simulink model "siWDqudong_FAN_MPC"  (R2024b)
settings: Solver=ode4  StartTime=0.0  StopTime=30  FixedStep=0.0005  RelTol=1e-3
undefined symbols (not defined in the file): MotorData, Q_beta_tune, Q_yaw_tune, R_alloc_tune, R_rate_tune, Road_Curvature_Map, Road_Mu_Map, Sim_Mu_Set, Sim_Vx_Set, Target_Speed_Map, W_util_tune
libraries: Solver_SF x1
(part 1 of 3)
Description:
  | V6 normalized model with fixed-speed PI torque demand. Created from V5; no implicit underspeed behavior in low-mu curves.
settings Model: SimulationMode=accelerator  Creator=zlm22  LastModifiedBy=zlm22
settings SolverCC: InsertRTBMode=Always
settings RTWCC: BuildConfiguration=Faster Runs

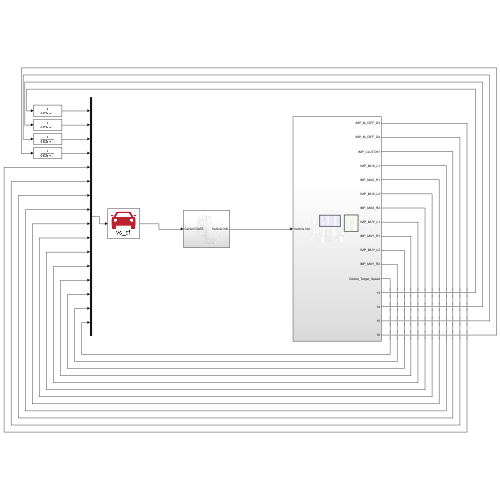
[thumbnail: Simulink's stored preview of the top-level diagram]
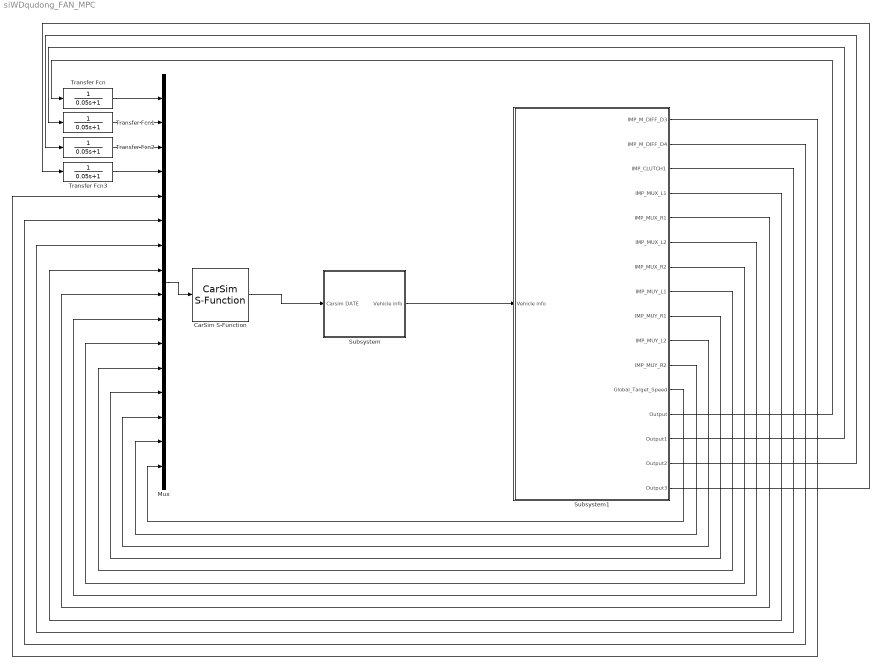
== system siWDqudong_FAN_MPC ==
  CarSim S-Function : Solver_SF/CarSim S-Function  Priority=1  SIMFILE=D:\Program Files (x86)\CarSim2024.1_DATA\simfile.sim  Run_RTs=off  vs_state_ind=Run  StopMode_ind=Vehicle Model
  Mux : Mux  Inputs=16
  Subsystem : Subsystem
  Subsystem1 : Subsystem
  Transfer Fcn{,1..3} (4 alike) : TransferFcn  Denominator=[0.05 1]
  wires:
  Transfer Fcn/1 -> Mux/1
  Transfer Fcn1/1 -> Mux/2
  Transfer Fcn2/1 -> Mux/3
  Transfer Fcn3/1 -> Mux/4
  Subsystem/1(Vehicle info) -> Subsystem1/1(Vehicle info)
  Subsystem1/1(IMP_M_DIFF_D3) -> Mux/5
  Subsystem1/2(IMP_M_DIFF_D4) -> Mux/6
  Subsystem1/3(IMP_CLUTCH1) -> Mux/7
  Subsystem1/4(IMP_MUX_L1) -> Mux/8
  Subsystem1/5(IMP_MUX_R1) -> Mux/9
  Subsystem1/6(IMP_MUX_L2) -> Mux/10
  Subsystem1/7(IMP_MUX_R2) -> Mux/11
  Subsystem1/8(IMP_MUY_L1) -> Mux/12
  Subsystem1/9(IMP_MUY_R1) -> Mux/13
  Subsystem1/10(IMP_MUY_L2) -> Mux/14
  Subsystem1/11(IMP_MUY_R2) -> Mux/15
  Subsystem1/12(Global_Target_Speed) -> Mux/16
  Subsystem1/13(Output) -> Transfer Fcn/1
  Subsystem1/14(Output1) -> Transfer Fcn1/1
  Subsystem1/15(Output2) -> Transfer Fcn2/1
  Subsystem1/16(Output3) -> Transfer Fcn3/1
  Mux/1 -> CarSim S-Function/1
  CarSim S-Function/1 -> Subsystem/1(Carsim DATE)

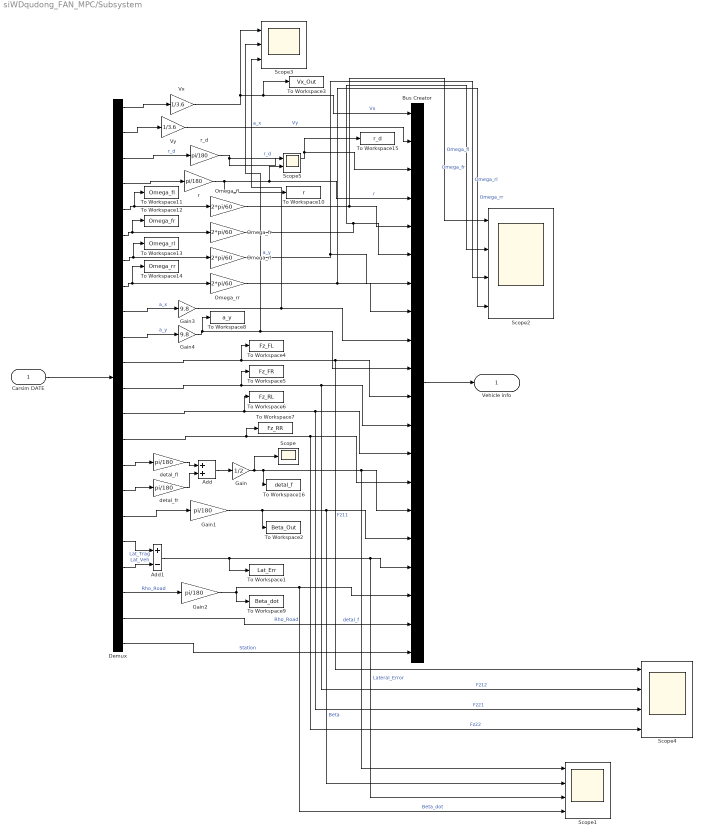
== system siWDqudong_FAN_MPC/Subsystem ==
  Carsim DATE : Inport
  Add : Sum
  Add1 : Sum  Inputs=+-
  Bus Creator : BusCreator  Inputs=20
  Demux : Demux  Outputs=22
  Gain : Gain  Gain=1/2
  Gain1 : Gain  Gain=pi/180
  Gain2 : Gain  Gain=pi/180
  Gain3 : Gain  Gain=9.8
  Gain4 : Gain  Gain=9.8
  Omega_fl : Gain  Gain=2*pi/60
  Omega_fr : Gain  Gain=2*pi/60
  Omega_rl : Gain  Gain=2*pi/60
  Omega_rr : Gain  Gain=2*pi/60
  Scope : Scope
  Scope1 : Scope  NumInputPorts=4
  Scope2 : Scope  NumInputPorts=4
  Scope3 : Scope  NumInputPorts=3
  Scope4 : Scope  NumInputPorts=4
  Scope5 : Scope  NumInputPorts=2
  To Workspace1 : ToWorkspace  VariableName=Lat_Err  SampleTime=-1
  To Workspace10 : ToWorkspace  VariableName=r  SampleTime=-1
  To Workspace11 : ToWorkspace  VariableName=Omega_fl  SampleTime=-1
  To Workspace12 : ToWorkspace  VariableName=Omega_fr  SampleTime=-1
  To Workspace13 : ToWorkspace  VariableName=Omega_rl  SampleTime=-1
  To Workspace14 : ToWorkspace  VariableName=Omega_rr  SampleTime=-1
  To Workspace15 : ToWorkspace  VariableName=r_d  SampleTime=-1
  To Workspace16 : ToWorkspace  VariableName=detal_f  SampleTime=-1
  To Workspace2 : ToWorkspace  VariableName=Beta_Out  SampleTime=-1
  To Workspace3 : ToWorkspace  VariableName=Vx_Out  SampleTime=-1
  To Workspace4 : ToWorkspace  VariableName=Fz_FL  SaveFormat=Timeseries  SampleTime=-1
  To Workspace5 : ToWorkspace  VariableName=Fz_FR  SaveFormat=Timeseries  SampleTime=-1
  To Workspace6 : ToWorkspace  VariableName=Fz_RL  SaveFormat=Timeseries  SampleTime=-1
  To Workspace7 : ToWorkspace  VariableName=Fz_RR  SaveFormat=Timeseries  SampleTime=-1
  To Workspace8 : ToWorkspace  VariableName=a_y  SampleTime=-1
  To Workspace9 : ToWorkspace  VariableName=Beta_dot  SampleTime=-1
  Vx : Gain  Gain=1/3.6
  Vy : Gain  Gain=1/3.6
  detal_fl : Gain  Gain=pi/180
  detal_fr : Gain  Gain=pi/180
  r : Gain  Gain=pi/180
  r_d : Gain  Gain=pi/180
  Vehicle info : Outport
  wires:
  Demux/3 -> r_d/1  "r_d"
  Demux/11 -> To Workspace4/1, Scope4/1, Bus Creator/11  "Fz11"
  Demux/8 -> To Workspace14/1, Omega_rr/1
  Vy/1 -> Bus Creator/2  "Vy"
  Demux/7 -> To Workspace13/1, Omega_rl/1
  Demux/14 -> To Workspace7/1, Scope4/4, Bus Creator/14  "Fz22"
  Demux/4 -> r/1
  Demux/5 -> To Workspace11/1, Omega_fl/1
  Demux/13 -> To Workspace6/1, Scope4/3, Bus Creator/13  "Fz21"
  Omega_rl/1 -> Scope2/3, Bus Creator/7  "Omega_rl"
  Demux/12 -> To Workspace5/1, Scope4/2, Bus Creator/12  "Fz12"
  Demux/16 -> detal_fr/1
  Omega_fr/1 -> Scope2/2, Bus Creator/6  "Omega_fr"
  Demux/6 -> To Workspace12/1, Omega_fr/1
  Demux/15 -> detal_fl/1
  Vx/1 -> Scope3/1, To Workspace3/1, Bus Creator/1  "Vx"
  r/1 -> Scope5/2, Bus Creator/4, To Workspace10/1  "r"
  Bus Creator/1 -> Vehicle info/1
  Omega_fl/1 -> Scope2/1, Bus Creator/5  "Omega_fl"
  Omega_rr/1 -> Scope2/4, Bus Creator/8  "Omega_rr"
  Demux/10 -> Gain4/1  "a_y"
  Demux/9 -> Gain3/1  "a_x"
  detal_fr/1 -> Add/2
  detal_fl/1 -> Add/1
  Add/1 -> Gain/1
  Gain/1 -> Scope/1, To Workspace16/1, Scope1/1, Bus Creator/15  "detal_f"
  Demux/1 -> Vx/1
  Demux/2 -> Vy/1
  Demux/17 -> Gain1/1
  Gain1/1 -> To Workspace2/1, Bus Creator/16, Scope1/2  "Beta"
  Gain2/1 -> Scope1/4, Bus Creator/18, To Workspace9/1  "Beta_dot"
  r_d/1 -> To Workspace15/1, Bus Creator/3, Scope5/1  "r_d"
  Carsim DATE/1 -> Demux/1
  Gain4/1 -> To Workspace8/1, Scope3/2, Bus Creator/10  "a_y"
  Gain3/1 -> Scope3/3, Bus Creator/9  "a_x"
  Demux/22 -> Bus Creator/20  "Station"
  Demux/21 -> Bus Creator/19  "Rho_Road"
  Demux/20 -> Gain2/1  "Rho_Road"
  Demux/18 -> Add1/1  "Lat_Trag"
  Demux/19 -> Add1/2  "Lat_Veh"
  Add1/1 -> To Workspace1/1, Scope1/3, Bus Creator/17  "Lateral_Error"

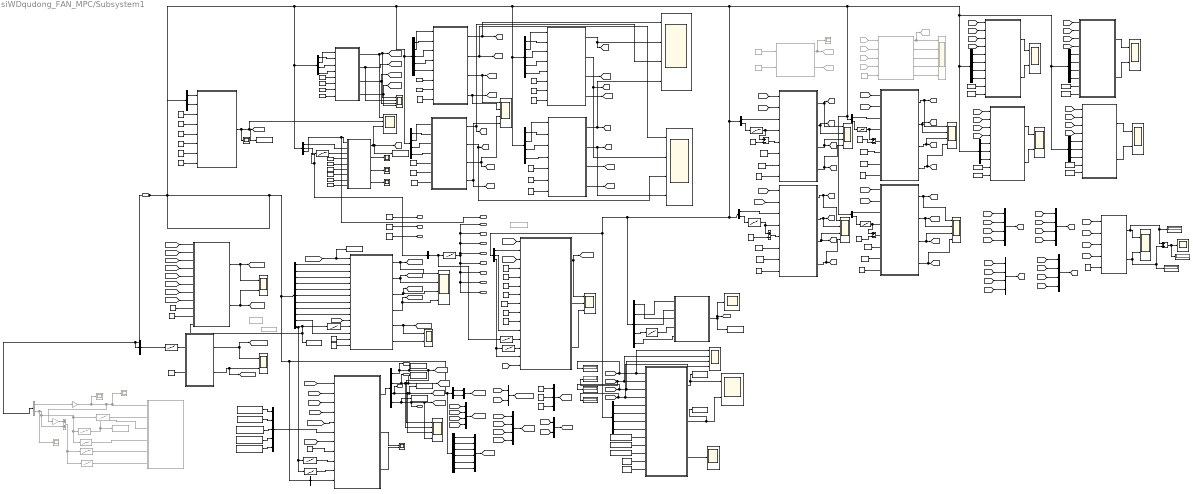
== system siWDqudong_FAN_MPC/Subsystem1 ==
  note: E_total_kWh
  note: Subsystem3
  note: 轮胎力
  Vehicle info : Inport
  Add1 : Sum
  Add{2..4,6} (4 alike) : Sum  Inputs=+-
  Add5 : Sum  Commented=on
  Bus Creator : BusCreator  Inputs=6
  Bus Creator1 : BusCreator  Inputs=2
  Bus Selector : BusSelector  OutputSignals=Omega_fl,Omega_fr,Omega_rl,Omega_rr,Fz11,Fz12,Fz21,Fz22,a_y,Lateral_Error,Station
  Bus Selector1 : BusSelector  OutputSignals=Vx,detal_f,Fz11,Fz12,Fz21,Fz22
  Bus Selector10 : BusSelector  OutputSignals=Fz11,Station
  Bus Selector11 : BusSelector  OutputSignals=Fz21,Station
  Bus Selector12 : BusSelector  OutputSignals=Fz12,Station
  Bus Selector13 : BusSelector  OutputSignals=Fz22,Station
  Bus Selector15 : BusSelector  Commented=on  OutputSignals=Vx,Station
  Bus Selector16 : BusSelector  OutputSignals=detal_f
  Bus Selector17 : BusSelector  OutputSignals=Vx,Vy,r_d,detal_f
  Bus Selector19 : BusSelector  OutputSignals=Vx,Vy,r_d,detal_f
  Bus Selector2 : BusSelector  OutputSignals=Beta,r_d
  Bus Selector20 : BusSelector  OutputSignals=Vx,Vy,r_d
  Bus Selector21 : BusSelector  OutputSignals=Vx,Vy,r_d
  Bus Selector22 : BusSelector  OutputSignals=Station
  Bus Selector23 : BusSelector  OutputSignals=detal_f,Station,Vx
  Bus Selector24 : BusSelector  OutputSignals=Station
  Bus Selector25 : BusSelector  OutputSignals=Omega_fl,Omega_fr,Omega_rl,Omega_rr
  Bus Selector26 : BusSelector  OutputSignals=Vx,detal_f,Beta
  Bus Selector27 : BusSelector  OutputSignals=Vx,Beta,Beta_dot,Station,detal_f
  Bus Selector3 : BusSelector  OutputSignals=Vx,detal_f
  Bus Selector5 : BusSelector  OutputSignals=Vy,Vx,r_d,Omega_fl,detal_f
  Bus Selector6 : BusSelector  OutputSignals=Vy,Vx,r_d,detal_f
  Bus Selector7 : BusSelector  OutputSignals=Vy,Vx,r_d,Omega_fr,detal_f
  Bus Selector8 : BusSelector  OutputSignals=Vy,Vx,r_d,Omega_rl
  Bus Selector9 : BusSelector  OutputSignals=Vy,Vx,r_d,Omega_rr
  Constant{1,7,18,21,30,48,90} (7 alike) : Constant  Value=1.152
  Constant{2,8,10,13,49,93,95} (7 alike) : Constant  Value=1.528
  Constant{9,11,14,16..17,19,78,92,94,96} (10 alike) : Constant  Value=1.565
  Constant{12,15,20,22,54} (5 alike) : Constant  Value=0.347
  Constant{23..25,60,82} (5 alike) : Constant  Value=0
  Constant{26,73,81,84,91} (5 alike) : Constant  Value=0.05
  Constant27 : Constant  Commented=on  Value=3
  Constant28 : Constant  Commented=on  Value=0.001
  Constant{29,32,35,38} (4 alike) : Constant  Value=0.6
  Constant{3,31,37,50,79} (5 alike) : Constant  Value=63833
  Constant33 : Constant  Value=44230
  Constant{4,34,40,51,88} (5 alike) : Constant  Value=48729
  Constant36 : Constant  Value=57917
  Constant39 : Constant  Value=44230
  Constant41 : Constant  Commented=on  Value=0.347
  Constant{6,42,59,86,97} (5 alike) : Constant  Value=0.01
  Constant43 : Constant  Value=800
  Constant44 : Constant  Commented=on  Value=Sim_Mu_Set
  Constant45 : Constant  Value=MotorData.Speed_Axis
  Constant47 : Constant  Value=1810
  Constant5 : Constant  Value=1810
  Constant52 : Constant  Value=9.81
  Constant53 : Constant  Value=MotorData.Torque_Axis
  Constant55 : Constant  Value=1810
  Constant56 : Constant  Value=9.81
  Constant57 : Constant  Value=45
  Constant58 : Constant  Value=5.0
  Constant63 : Constant  Value=Q_beta_tune
  Constant64 : Constant  Value=Q_yaw_tune
  Constant66 : Constant  Commented=on  Value=Sim_Vx_Set
  Constant68 : Constant  Commented=on  Value=Sim_Vx_Set
  Constant69 : Constant  Value=R_alloc_tune
  Constant71 : Constant  Value=R_rate_tune
  Constant72 : Constant  Value=W_util_tune
  Constant77 : Constant  Value=MotorData.Eff_Map
  Constant80 : Constant  Value=0.005
  Constant89 : Constant  Value=57917
  Demux : Demux
  Display{,1..6} (7 alike) : Display
  From68 : From  Commented=on  GotoTag=Fx_fl
  From69 : From  Commented=on  GotoTag=Fx_fr
  From70 : From  Commented=on  GotoTag=Fx_rl
  From71 : From  Commented=on  GotoTag=Fx_rr
  Gain : Gain  Commented=on  Gain=3.6
  Gain2 : Gain  Commented=on  Gain=1.2
  Goto29 : Goto  Commented=on  GotoTag=mu_y
  Goto5 : Goto  Commented=on  GotoTag=mu_x
  MATLAB Function : MATLAB Function  TreatAsAtomicUnit=on  SystemSampleTime=0.01
  MATLAB Function1 : MATLAB Function  TreatAsAtomicUnit=on
  MATLAB Function10 : MATLAB Function  TreatAsAtomicUnit=on
  MATLAB Function14 : MATLAB Function  Commented=on  TreatAsAtomicUnit=on
  MATLAB Function15 : MATLAB Function  TreatAsAtomicUnit=on  SystemSampleTime=0.01
  MATLAB Function16 : MATLAB Function  TreatAsAtomicUnit=on
  MATLAB Function17 : MATLAB Function  TreatAsAtomicUnit=on
  MATLAB Function18 : MATLAB Function  TreatAsAtomicUnit=on
  MATLAB Function19 : MATLAB Function  TreatAsAtomicUnit=on  SystemSampleTime=0.01
  MATLAB Function2 : MATLAB Function  TreatAsAtomicUnit=on  SystemSampleTime=0.01
  MATLAB Function20 : MATLAB Function  Commented=on  TreatAsAtomicUnit=on
  MATLAB Function21 : MATLAB Function  TreatAsAtomicUnit=on  SystemSampleTime=0.01
  MATLAB Function22 : MATLAB Function  TreatAsAtomicUnit=on
  MATLAB Function23 : MATLAB Function  TreatAsAtomicUnit=on  SystemSampleTime=0.01
  MATLAB Function24 : MATLAB Function  TreatAsAtomicUnit=on
  MATLAB Function25 : MATLAB Function  TreatAsAtomicUnit=on
  MATLAB Function3 : MATLAB Function  TreatAsAtomicUnit=on  SystemSampleTime=0.01
  MATLAB Function4 : MATLAB Function  TreatAsAtomicUnit=on
  MATLAB Function5 : MATLAB Function  TreatAsAtomicUnit=on
  MATLAB Function6 : MATLAB Function  TreatAsAtomicUnit=on
  MATLAB Function7 : MATLAB Function  TreatAsAtomicUnit=on
  MATLAB Function8 : MATLAB Function  TreatAsAtomicUnit=on
  MATLAB Function9 : MATLAB Function  TreatAsAtomicUnit=on
  MU : Lookup_n-D  Commented=on  NumberOfTableDimensions=1  BreakpointsForDimension1=Road_Mu_Map(:, 1)  Table=Road_Mu_Map(:, 2)  InternalRulePriority=Speed  RndMeth=Simplest
  Mu12 : Lookup_n-D  Commented=on  NumberOfTableDimensions=1  BreakpointsForDimension1=Road_Mu_Map(:, 1)  Table=Road_Mu_Map(:, 2)  InternalRulePriority=Speed  RndMeth=Simplest
  Mu{2..9,13..14} (10 alike) : Lookup_n-D  NumberOfTableDimensions=1  BreakpointsForDimension1=Road_Mu_Map(:, 1)  Table=Road_Mu_Map(:, 2)  InternalRulePriority=Speed  RndMeth=Simplest
  Mux : Mux  Inputs=2
  Mux{1,5..9} (6 alike) : Mux
  Mux10 : Mux  Inputs=5
  Mux2 : Mux  Inputs=2
  Mux4 : Mux  Inputs=3
  Radius1 : Lookup_n-D  Commented=on  NumberOfTableDimensions=1  BreakpointsForDimension1=Road_Curvature_Map(:, 1)  Table=Road_Curvature_Map(:, 2)  InternalRulePriority=Speed  RndMeth=Simplest
  Radius2 : Lookup_n-D  Commented=on  NumberOfTableDimensions=1  BreakpointsForDimension1=Road_Curvature_Map(:, 1)  Table=Road_Curvature_Map(:, 2)  InternalRulePriority=Speed  RndMeth=Simplest
  Radius3 : Lookup_n-D  NumberOfTableDimensions=1  BreakpointsForDimension1=Road_Curvature_Map(:, 1)  Table=Road_Curvature_Map(:, 2)  InternalRulePriority=Speed  RndMeth=Simplest
  Radius4 : Lookup_n-D  NumberOfTableDimensions=1  BreakpointsForDimension1=Road_Curvature_Map(:, 1)  Table=Road_Curvature_Map(:, 2)  InternalRulePriority=Speed  RndMeth=Simplest
  SI : Scope
  Scope{,1..2,5,10..14,45} (10 alike) : Scope  NumInputPorts=2
  Scope{3..4,6,9,15..18,20,28,30,48} (12 alike) : Scope  NumInputPorts=4
  Scope{8,21..22,47} (4 alike) : Scope  Commented=on
  Scope{23,32..34,44,49} (6 alike) : Scope
  Scope24 : Scope  Commented=on  NumInputPorts=5
  Scope7 : Scope  NumInputPorts=3
  T_max : Constant  Value=800
  T_min : Constant  Value=-200
  To Workspace : ToWorkspace  VariableName=SI_Out  SaveFormat=Timeseries  SampleTime=-1
  To Workspace10 : ToWorkspace  VariableName=R_ref  SampleTime=-1
  To Workspace12 : ToWorkspace  VariableName=beta_ref  SampleTime=-1
  To Workspace13 : ToWorkspace  VariableName=Sim_Station  SampleTime=-1
  To Workspace14 : ToWorkspace  Commented=on  VariableName=Mu  SampleTime=-1
  To Workspace3 : ToWorkspace  VariableName=Total_Power_Out  SampleTime=-1
  To Workspace4 : ToWorkspace  VariableName=Motor_Torque_FL  SampleTime=-1
  To Workspace5 : ToWorkspace  VariableName=Motor_Torque_FR  SampleTime=-1
  To Workspace6 : ToWorkspace  VariableName=Motor_Torque_RL  SampleTime=-1
  To Workspace7 : ToWorkspace  VariableName=Motor_Torque_RR  SampleTime=-1
  To Workspace8 : ToWorkspace  VariableName=E_total_kWh  SampleTime=-1
  To Workspace9 : ToWorkspace  VariableName=P_total_kW  SampleTime=-1
  Vx1 : Lookup_n-D  NumberOfTableDimensions=1  BreakpointsForDimension1=Target_Speed_Map(:, 1)  Table=Target_Speed_Map(:, 2)  InternalRulePriority=Speed  RndMeth=Simplest
  Vx2 : Lookup_n-D  Commented=on  NumberOfTableDimensions=1  BreakpointsForDimension1=Target_Speed_Map(:, 1)  Table=Target_Speed_Map(:, 2)  InternalRulePriority=Speed  RndMeth=Simplest
  delta_T_max : Constant  Value=2000
  unitire轮胎力 : MATLAB Function  TreatAsAtomicUnit=on
  侧偏角计算 : MATLAB Function  TreatAsAtomicUnit=on
  总需求扭矩 : Goto  Commented=on  GotoTag=Td
  横纵向附着系数 : MATLAB Function  Commented=on  TreatAsAtomicUnit=on
  IMP_M_DIFF_D3 : Outport
  IMP_M_DIFF_D4 : Outport  Port=2
  IMP_CLUTCH1 : Outport  Port=3
  IMP_MUX_L1 : Outport  Port=4
  IMP_MUX_R1 : Outport  Port=5
  IMP_MUX_L2 : Outport  Port=6
  IMP_MUX_R2 : Outport  Port=7
  IMP_MUY_L1 : Outport  Port=8
  IMP_MUY_R1 : Outport  Port=9
  IMP_MUY_L2 : Outport  Port=10
  IMP_MUY_R2 : Outport  Port=11
  Global_Target_Speed : Outport  Port=12
  Output : Outport  Port=13
  Output1 : Outport  Port=14
  Output2 : Outport  Port=15
  Output3 : Outport  Port=16
  wires:
  MATLAB Function5/1(Sx_fr) -> [Sx_fr], Scope9/2
  Bus Selector7/1 -> MATLAB Function5/2(Vy)  "<Vy>"
  Constant13/1 -> MATLAB Function7/5(lr)
  Constant21/1 -> MATLAB Function5/6(lf)
  MATLAB Function8/3(Fbar_x_rl) -> Scope17/3, [Fsx_rl]
  MATLAB Function6/1(Sx_rl) -> [Sx_rl], Scope9/3
  Constant14/1 -> MATLAB Function7/6(twr)
  MATLAB Function7/1(Sx_rr) -> [Sx_rr], Scope9/4
  Constant1/1 -> MATLAB Function4/3(lf)
  Bus Selector11/1 -> MATLAB Function8/3(Fz_rl)  "<Fz21>"
  MATLAB Function9/2(Fy_fr) -> Scope15/2, [Fy_fr]
  Bus Selector6/4 -> 侧偏角计算/4(delta_f_rad)  "<detal_f>"
  MATLAB Function5/2(Sy_fr) -> [Sy_fr], Scope28/2
  Constant47/1 -> MATLAB Function17/4(m)
  Bus Selector5/5 -> unitire轮胎力/5(delta_f)  "<detal_f>"
  [Sx_fr] -> MATLAB Function9/1(Sx_fr)
  Constant52/1 -> MATLAB Function17/9(g)
  MATLAB Function17/1(r_d) -> [r_d], To Workspace10/1, Scope30/3  "r_ref"
  Constant15/1 -> MATLAB Function7/7(Re)
  MATLAB Function9/1(Fx_fr) -> Scope15/1, [Fx_fr]
  MATLAB Function10/1(Fx_rr) -> Scope18/1, [Fx_rr]
  MATLAB Function1/1(Fx_fl) -> [Fx_fl], Scope48/1
  MATLAB Function7/2(Sy_rr) -> Scope28/4, [Sy_rr]
  Constant2/1 -> MATLAB Function4/4(lr)
  MATLAB Function20/1(Td) -> Scope24/1, 总需求扭矩/1
  Constant38/1 -> MATLAB Function10/8(E)
  [Sy_fr] -> MATLAB Function9/2(Sy_fr)
  Constant9/1 -> 侧偏角计算/7(twf)
  Bus Selector10/1 -> MATLAB Function1/3(Fz_fl)  "<Fz11>"
  Bus Selector7/4 -> MATLAB Function5/4(omega_fr)  "<Omega_fr>"
  Constant4/1 -> MATLAB Function4/6(Kyr)
  Constant5/1 -> MATLAB Function4/7(m)
  Constant8/1 -> 侧偏角计算/6(lr)
  Constant27/1 -> 横纵向附着系数/1(road_condition)
  Bus Selector3/2 -> MATLAB Function4/2(delta_f)  "<detal_f>"
  Bus Selector3/1 -> MATLAB Function4/1(Vx)  "<Vx>"
  Constant6/1 -> MATLAB Function4/8(dt)
  Constant17/1 -> MATLAB Function5/7(twf)
  MATLAB Function4/1(beta_ref) -> Scope44/1, To Workspace12/1, [beta_ref], Scope30/2  "beta_ref"
  MATLAB Function1/3(Fbar_x_fl) -> Scope48/3, [Fsx_fl]
  Constant48/1 -> MATLAB Function17/5(lf)
  Constant3/1 -> MATLAB Function4/5(Kyf)
  MATLAB Function1/4(Fbar_y_fl) -> Scope48/4, [Fsy_fl]
  Constant29/1 -> MATLAB Function1/8(E)
  From68/1 -> MATLAB Function20/1(Fx_fl)
  Bus Selector8/4 -> MATLAB Function6/4(omega_rl)  "<Omega_rl>"
  MATLAB Function6/2(Sy_rl) -> Scope28/3, [Sy_rl]
  From71/1 -> MATLAB Function20/4(Fx_rr)
  Constant50/1 -> MATLAB Function17/7(Kf0)
  Bus Selector5/4 -> unitire轮胎力/4(omega_fl)  "<Omega_fl>"
  Bus Selector6/1 -> 侧偏角计算/2(Vy)  "<Vy>"
  Constant49/1 -> MATLAB Function17/6(lr)
  MATLAB Function8/4(Fbar_y_rl) -> Scope17/4, [Fsy_rl]
  MATLAB Function9/4(Fbar_y_fr) -> Scope15/4, [Fsy_fr]
  Constant51/1 -> MATLAB Function17/8(Kr0)
  MATLAB Function17/4(r_limit) -> Scope34/1
  MATLAB Function17/2(K_s) -> Scope32/1
  MATLAB Function17/3(r_ideal) -> Scope33/1
  Constant22/1 -> MATLAB Function5/8(Re)
  横纵向附着系数/1(mu_x) -> Scope47/1, Goto5/1
  Bus Selector12/1 -> MATLAB Function9/3(Fz_fr)  "<Fz12>"
  [Sx_fl] -> MATLAB Function1/1(Sx_fl)
  Bus Selector9/4 -> MATLAB Function7/4(omega_rr)  "<Omega_rr>"
  unitire轮胎力/1(Sx_fl) -> Scope9/1, [Sx_fl]
  From69/1 -> MATLAB Function20/2(Fx_fr)
  From70/1 -> MATLAB Function20/3(Fx_rl)
  Constant10/1 -> MATLAB Function6/5(lr)
  [Sy_rr] -> MATLAB Function10/2(Sy_rr)
  Constant41/1 -> MATLAB Function20/5(r_e)
  Constant35/1 -> MATLAB Function9/8(E)
  [Sy_rl] -> MATLAB Function8/2(Sy_rl)
  Constant7/1 -> 侧偏角计算/5(lf)
  MATLAB Function9/3(Fbar_x_fr) -> Scope15/3, [Fsx_fr]
  Bus Selector13/1 -> MATLAB Function10/3(Fz_rr)  "<Fz22>"
  MATLAB Function1/2(Fy_fl) -> [Fy_fl], Scope48/2
  MATLAB Function10/4(Fbar_y_rr) -> Scope18/4, [Fsy_rr]
  MATLAB Function10/2(Fy_rr) -> Scope18/2, [Fy_rr]
  MATLAB Function10/3(Fbar_x_rr) -> Scope18/3, [Fsx_rr]
  Mu5/1 -> Add6/1, MATLAB Function1/4(mu_x)
  [Sx_rr] -> MATLAB Function10/1(Sx_rr)
  Constant32/1 -> MATLAB Function8/8(E)
  MATLAB Function8/1(Fx_rl) -> Scope17/1, [Fx_rl]
  MATLAB Function8/2(Fy_rl) -> Scope17/2, [Fy_rl]
  [Sy_fl] -> MATLAB Function1/2(Sy_fl)
  Constant19/1 -> unitire轮胎力/7(twf)
  [Sx_rl] -> MATLAB Function8/1(Sx_rl)
  横纵向附着系数/2(mu_y) -> Goto29/1
  Constant28/1 -> 横纵向附着系数/2(slip_ratio)
  Bus Selector9/1 -> MATLAB Function7/2(Vy)  "<Vy>"
  Constant18/1 -> unitire轮胎力/6(lf)
  unitire轮胎力/2(Sy_fl) -> Scope28/1, [Sy_fl]
  Constant16/1 -> 侧偏角计算/8(twr)
  Constant11/1 -> MATLAB Function6/6(twr)
  Bus Selector8/1 -> MATLAB Function6/2(Vy)  "<Vy>"
  Constant20/1 -> unitire轮胎力/8(Re)
  Bus Selector5/1 -> unitire轮胎力/2(Vy)  "<Vy>"
  Vehicle info/1 -> Bus Selector/1, Bus Selector2/1, Bus Selector1/1, Bus Selector16/1, Bus Selector23/1, Bus Selector6/1, Bus Selector9/1, Bus Selector7/1, Bus Selector10/1, Bus Selector27/1, Bus Selector25/1, Bus Selector26/1, Bus Selector11/1, Bus Selector21/1, Bus Selector19/1, Bus Selector20/1, Bus Selector17/1, Bus Selector13/1, Bus Selector12/1, Bus Selector8/1, Bus Selector5/1, Bus Selector3/1, Bus Selector15/1, Bus Selector24/1
  MATLAB Function20/5(T_rr) -> Scope24/5
  MATLAB Function20/4(T_rl) -> Scope24/4
  MATLAB Function20/3(T_fr) -> Scope24/3
  MATLAB Function20/2(T_fl) -> Scope24/2
  [T_ZY_RR] -> Display3/1, MATLAB Function2/4(T_rr), Scope6/4
  [T_ZY_RL] -> Display2/1, Scope6/3, MATLAB Function2/3(T_rl)
  [T_ZY_FL] -> Display/1, MATLAB Function2/1(T_fl), Scope6/1
  [T_ZY_FR] -> Display1/1, MATLAB Function2/2(T_fr), Scope6/2
  Bus Selector25/1 -> MATLAB Function2/5(w_fl)  "<Omega_fl>"
  Bus Selector25/2 -> MATLAB Function2/6(w_fr)  "<Omega_fr>"
  Bus Selector25/3 -> MATLAB Function2/7(w_rl)  "<Omega_rl>"
  MATLAB Function2/3(P_avg_kW) -> Scope49/1
  Constant55/1 -> MATLAB Function15/4(m)
  Constant56/1 -> MATLAB Function15/5(g)
  MATLAB Function15/1(T_total) -> [T_total], Scope7/1
  MATLAB Function18/1(Vx_safe_cmd) -> Scope45/1, [Vx_safe_cmd]
  MATLAB Function18/2(Ax_cmd_final) -> Scope45/2, [Ax_cmd_final]
  [Vx_safe_cmd] -> MATLAB Function15/1(Vx_cmd)
  [Ax_cmd_final] -> MATLAB Function15/3(Ax_cmd)
  MATLAB Function2/2(E_total_kWh) -> To Workspace8/1, Scope2/2
  MATLAB Function2/1(P_total_kW) -> To Workspace9/1, Scope2/1
  Constant73/1 -> MATLAB Function18/2(dt)
  Bus Selector27/3 -> MATLAB Function19/2(Beta_dot)  "<Beta_dot>"
  MATLAB Function19/1(SI_Out) -> To Workspace/1, SI/1, [SI]  "SI_Out"
  [Fy_fl] -> MATLAB Function23/1(Fy_fl)
  [Fy_fr] -> MATLAB Function23/2(Fy_fr)
  [Fy_rl] -> MATLAB Function23/3(Fy_rl)
  [Fy_rr] -> MATLAB Function23/4(Fy_rr)
  [alpha_fl] -> MATLAB Function23/5(Alpha_fl)
  [alpha_fr] -> MATLAB Function23/6(Alpha_fr)
  [alpha_rl] -> MATLAB Function23/7(Alpha_rl)
  [alpha_rr] -> MATLAB Function23/8(Alpha_rr)
  Constant88/1 -> MATLAB Function23/10(Cr0)
  Constant79/1 -> MATLAB Function23/9(Cf0)
  MATLAB Function23/1(Cf_eq) -> Scope5/1, [Cf_eq]
  MATLAB Function23/2(Cr_eq) -> Scope5/2, [Cr_eq]
  Constant23/1 -> IMP_M_DIFF_D3/1
  Constant24/1 -> IMP_M_DIFF_D4/1
  Constant25/1 -> IMP_CLUTCH1/1
  Mu3/1 -> IMP_MUX_R2/1, IMP_MUX_L2/1, IMP_MUX_R1/1, IMP_MUX_L1/1, IMP_MUY_L1/1, IMP_MUY_R1/1, IMP_MUY_L2/1, IMP_MUY_R2/1
  Constant81/1 -> Add2/2
  Constant84/1 -> Add3/2
  Add4/1 -> MATLAB Function8/5(mu_y)
  Mu7/1 -> MATLAB Function8/4(mu_x), Add4/1
  Constant91/1 -> Add4/2
  [T_total] -> To Workspace3/1, MATLAB Function3/1(T_total_req)
  Bus Selector/8 -> MATLAB Function3/9(Fz_rr)  "<Fz22>"
  Bus Selector/7 -> MATLAB Function3/8(Fz_rl)  "<Fz21>"
  Bus Selector/6 -> MATLAB Function3/7(Fz_fr)  "<Fz12>"
  Bus Selector/5 -> MATLAB Function3/6(Fz_fl)  "<Fz11>"
  Bus Selector/4 -> MATLAB Function3/5(w_rr)  "<Omega_rr>"
  Bus Selector/3 -> MATLAB Function3/4(w_rl)  "<Omega_rl>"
  Bus Selector/2 -> MATLAB Function3/3(w_fr)  "<Omega_fr>"
  Bus Selector/1 -> MATLAB Function3/2(w_fl)  "<Omega_fl>"
  Constant43/1 -> MATLAB Function3/14(T_motor_max)
  MATLAB Function3/5(Mode_Out) -> Scope/1, [Mode_Signal]
  MATLAB Function3/1(T_ref_fl) -> [T_ref_fl], Scope4/1
  MATLAB Function3/2(T_ref_fr) -> [T_ref_fr], Scope4/2
  MATLAB Function3/3(T_ref_rl) -> [T_ref_rl], Scope4/3
  MATLAB Function3/4(T_ref_rr) -> [T_ref_rr], Scope4/4
  Constant42/1 -> MATLAB Function3/15(dt)
  [beta_ref] -> Mux/1
  [r_d] -> Mux/2
  [T_ref_fl] -> Mux1/1
  [T_ref_fr] -> Mux1/2
  [T_ref_rl] -> Mux1/3
  [T_ref_rr] -> Mux1/4
  Mux1/1 -> [T_ref_upper]
  [Cf_eq] -> Mux2/1
  [Cr_eq] -> Mux2/2
  Mux2/1 -> [Stiffness_Input]
  Bus Selector1/3 -> Bus Creator/3  "<Fz11>"
  Bus Selector1/4 -> Bus Creator/4  "<Fz12>"
  Bus Selector1/5 -> Bus Creator/5  "<Fz21>"
  Bus Selector1/6 -> Bus Creator/6  "<Fz22>"
  Bus Creator/1 -> [Vehicle_State]
  Bus Selector2/1 -> Bus Creator1/1  "<Beta>"
  Bus Selector2/2 -> Bus Creator1/2  "<r_d>"
  Bus Creator1/1 -> [x_curr]
  T_min/1 -> Mux4/1
  T_max/1 -> Mux4/2
  delta_T_max/1 -> Mux4/3
  Mux4/1 -> [Constraints]
  [x_curr] -> MATLAB Function/1(x_curr)
  [x_ref] -> MATLAB Function/2(x_ref)
  [T_ref_upper] -> MATLAB Function/3(T_ref_upper_in)
  [Vehicle_State] -> MATLAB Function/4(Vehicle_State)
  [Stiffness_Input] -> MATLAB Function/5(Stiffness_Input)
  [Constraints] -> MATLAB Function/7(Constraints)
  MATLAB Function/2(Solver_Status) -> Scope1/1
  MATLAB Function/3(Debug_Info) -> Scope1/2
  MATLAB Function/1(T_final_opt) -> Demux/1
  Demux/1 -> Output/1, To Workspace4/1, [T_ZY_FL], Scope3/1  "F11"
  Demux/2 -> Output1/1, To Workspace5/1, [T_ZY_FR], Scope3/2  "F12"
  Demux/3 -> Output2/1, To Workspace6/1, [T_ZY_RL], Scope3/3  "F21"
  Demux/4 -> To Workspace7/1, Output3/1, Scope3/4, [T_ZY_RR]  "F22"
  Constant54/1 -> MATLAB Function15/6(r_e)
  Constant60/1 -> MATLAB Function15/10(is_reset)
  Constant58/1 -> MATLAB Function15/8(Ki)
  Constant57/1 -> MATLAB Function15/7(Kp)
  Constant59/1 -> MATLAB Function15/9(dt)
  MATLAB Function15/2(T_ff) -> Scope7/2
  MATLAB Function15/3(T_fb) -> Scope7/3
  [alpha_fl] -> Mux5/1
  [alpha_fr] -> Mux5/2
  [alpha_rl] -> Mux5/3
  [alpha_rr] -> Mux5/4
  Mux5/1 -> [SlipAngles_in]
  Bus Selector/9 -> MATLAB Function3/10(Ay_in)  "<a_y>"
  [SI] -> MATLAB Function3/11(SI_in)
  Mu2/1 -> MATLAB Function3/12(Mu_in)
  Mu4/1 -> MATLAB Function17/3(mu)
  Mu9/1 -> MATLAB Function19/4(mu)
  Bus Selector25/4 -> MATLAB Function2/8(w_rr)  "<Omega_rr>"
  Constant45/1 -> MATLAB Function2/9(Map_Spd)
  Constant53/1 -> MATLAB Function2/10(Map_Trq)
  Constant77/1 -> MATLAB Function2/11(Map_Eff)
  Constant80/1 -> MATLAB Function2/12(dt)
  Constant82/1 -> MATLAB Function2/13(is_reset)
  Constant86/1 -> MATLAB Function/8(dt_in)
  Bus Selector/10 -> MATLAB Function3/13(Lat_Error_in)  "<Lateral_Error>"
  侧偏角计算/1(alpha_fl) -> Scope20/1, [alpha_fl], Scope30/1  "alpha_fl"
  侧偏角计算/2(alpha_fr) -> [alpha_fr], Scope20/2  "alpha_fr"
  侧偏角计算/3(alpha_rl) -> [alpha_rl], Scope20/3  "alpha_rl"
  侧偏角计算/4(alpha_rr) -> [alpha_rr], Scope20/4  "alpha_rr"
  Constant12/1 -> MATLAB Function6/7(Re)
  Bus Selector7/5 -> MATLAB Function5/5(delta_f)  "<detal_f>"
  Bus Selector5/3 -> unitire轮胎力/3(r)  "<r_d>"
  Bus Selector7/3 -> MATLAB Function5/3(r)  "<r_d>"
  Bus Selector8/3 -> MATLAB Function6/3(r)  "<r_d>"
  Bus Selector9/3 -> MATLAB Function7/3(r)  "<r_d>"
  Constant26/1 -> Add6/2
  Add6/1 -> MATLAB Function1/5(mu_y)
  Constant89/1 -> MATLAB Function1/6(Kx)
  Constant31/1 -> MATLAB Function1/7(Ky)
  Mu6/1 -> MATLAB Function9/4(mu_x), Add2/1
  Add2/1 -> MATLAB Function9/5(mu_y)
  Constant36/1 -> MATLAB Function9/6(Kx)
  Constant37/1 -> MATLAB Function9/7(Ky)
  Constant33/1 -> MATLAB Function8/6(Kx)
  Constant34/1 -> MATLAB Function8/7(Ky)
  Add3/1 -> MATLAB Function10/5(mu_y)
  Mu8/1 -> Add3/1, MATLAB Function10/4(mu_x)
  Constant39/1 -> MATLAB Function10/6(Kx)
  Constant40/1 -> MATLAB Function10/7(Ky)
  unitire轮胎力/3(Vsx_fl) -> Scope16/1, [Vsx_fl]
  unitire轮胎力/4(Vsy_fl) -> Scope16/2, [Vsy_fl]
  MATLAB Function6/3(Vsx_rl) -> [Vsx_rl], Scope16/3
  MATLAB Function6/4(Vsy_rl) -> [Vsy_rl], Scope16/4
  MATLAB Function7/3(Vsx_rr) -> [Vsx_rr]
  MATLAB Function7/4(Vsy_rr) -> [Vsy_rr]
  Bus Selector17/4 -> MATLAB Function16/8(delta_f)  "<detal_f>"
  Bus Selector17/3 -> MATLAB Function16/7(r)  "<r_d>"
  Bus Selector17/2 -> MATLAB Function16/6(Vy)  "<Vy>"
  Bus Selector17/1 -> MATLAB Function16/5(Vx)  "<Vx>"
  [Fx_fl] -> MATLAB Function16/1(Fx_fl)
  [Fy_fl] -> MATLAB Function16/2(Fy_fl)
  [Sx_fl] -> MATLAB Function16/3(Sx_fl)
  [Sy_fl] -> MATLAB Function16/4(Sy_fl)
  Constant30/1 -> MATLAB Function16/9(lf)
  Constant78/1 -> MATLAB Function16/10(twf)
  Constant92/1 -> MATLAB Function22/10(twf)
  Constant90/1 -> MATLAB Function22/9(lf)
  [Sy_fr] -> MATLAB Function22/4(Sy_fr)
  [Sx_fr] -> MATLAB Function22/3(Sx_fr)
  [Fx_fr] -> MATLAB Function22/2(Fy_fr)
  [Fx_fr] -> MATLAB Function22/1(Fx_fr)
  Bus Selector19/1 -> MATLAB Function22/5(Vx)  "<Vx>"
  Bus Selector19/2 -> MATLAB Function22/6(Vy)  "<Vy>"
  Bus Selector19/3 -> MATLAB Function22/7(r)  "<r_d>"
  Bus Selector19/4 -> MATLAB Function22/8(delta_f)  "<detal_f>"
  MATLAB Function16/1(Px_fl) -> Scope10/1
  MATLAB Function16/2(Py_fl) -> Scope10/2
  MATLAB Function22/1(Px_fr) -> Scope11/1
  MATLAB Function22/2(Py_fr) -> Scope11/2
  MATLAB Function24/2(Py_rl) -> Scope12/2
  MATLAB Function24/1(Px_rl) -> Scope12/1
  Bus Selector20/3 -> MATLAB Function24/7(r)  "<r_d>"
  Bus Selector20/2 -> MATLAB Function24/6(Vy)  "<Vy>"
  Bus Selector20/1 -> MATLAB Function24/5(Vx)  "<Vx>"
  [Fx_rl] -> MATLAB Function24/1(Fx_rl)
  [Fy_rl] -> MATLAB Function24/2(Fy_rl)
  [Sx_rl] -> MATLAB Function24/3(Sx_rl)
  [Sy_rl] -> MATLAB Function24/4(Sy_rl)
  Constant94/1 -> MATLAB Function24/9(twr)
  Constant93/1 -> MATLAB Function24/8(lr)
  Constant95/1 -> MATLAB Function25/8(lr)
  Constant96/1 -> MATLAB Function25/9(twr)
  [Sy_rr] -> MATLAB Function25/4(Sy_rr)
  [Sx_rr] -> MATLAB Function25/3(Sx_rr)
  [Fy_rr] -> MATLAB Function25/2(Fy_rr)
  [Fx_rr] -> MATLAB Function25/1(Fx_rr)
  Bus Selector21/1 -> MATLAB Function25/5(Vx)  "<Vx>"
  Bus Selector21/2 -> MATLAB Function25/6(Vy)  "<Vy>"
  Bus Selector21/3 -> MATLAB Function25/7(r)  "<r_d>"
  MATLAB Function25/1(Px_rr) -> Scope13/1
  MATLAB Function25/2(Py_rr) -> Scope13/2
  [Fx_fl] -> Mux6/1
  [Fx_fr] -> Mux6/2
  [Fx_rl] -> Mux6/3
  [Fx_rr] -> Mux6/4
  Mux6/1 -> [Fx]
  Mux7/1 -> [Fy]
  [Fy_rr] -> Mux7/4
  [Fy_rl] -> Mux7/3
  [Fy_fr] -> Mux7/2
  [Fy_fl] -> Mux7/1
  [Vsx_fl] -> Mux8/1
  [Vsx_fr] -> Mux8/2
  [Fy_rl] -> Mux8/3
  [Fy_rr] -> Mux8/4
  Mux8/1 -> [Vsy]
  MATLAB Function5/3(Vsx_fr) -> [Vsx_fr]
  MATLAB Function5/4(Vsy_fr) -> [Vsy_fr]
  Mux9/1 -> [Vsx]
  [Fy_rr] -> Mux9/4
  [Fy_rl] -> Mux9/3
  [Vsx_fr] -> Mux9/2
  [Vsy_fl] -> Mux9/1
  MATLAB Function21/2(E_lat_total) -> Add1/2, Display4/1, Scope14/2
  MATLAB Function21/1(E_long_total) -> Add1/1, Display6/1, Scope14/1
  [Fx] -> MATLAB Function21/1(Fx)
  [Fy] -> MATLAB Function21/2(Fy)
  [Vsx] -> MATLAB Function21/3(Vsx)
  [Vsy] -> MATLAB Function21/4(Vsy)
  Constant97/1 -> MATLAB Function21/5(dt)
  Mux/1 -> [x_ref]
  MATLAB Function3/6(Debug_Info) -> Scope/2
  Bus Selector23/1 -> MATLAB Function17/2(delta_f)  "<detal_f>"
  Bus Selector6/3 -> 侧偏角计算/3(r)  "<r_d>"
  Bus Selector/11 -> MATLAB Function23/11(Mu_Current), To Workspace13/1, Mu2/1, Radius3/1, Mu13/1  "<Station>"
  Bus Selector22/1 -> Mu3/1, Mu14/1  "<Station>"
  Bus Selector23/2 -> Bus Selector22/1, Mu4/1  "<Station>"
  Bus Selector10/2 -> Mu5/1  "<Station>"
  Bus Selector12/2 -> Mu6/1  "<Station>"
  Bus Selector11/2 -> Mu7/1  "<Station>"
  Bus Selector13/2 -> Mu8/1  "<Station>"
  Bus Selector27/4 -> Mu9/1  "<Station>"
  Add1/1 -> Display5/1, Scope23/1
  Bus Selector6/2 -> 侧偏角计算/1(Vx)  "<Vx>"
  Bus Selector27/1 -> MATLAB Function19/3(Vx)  "<Vx>"
  Bus Selector24/1 -> Vx1/1  "<Station>"
  Bus Selector23/3 -> Global_Target_Speed/1, MATLAB Function17/1(Vx)  "<Vx>"
  Bus Selector15/2 -> Scope8/1, Vx2/1, MU/1, Radius1/1, Add5/2  "<Station>"
  MU/1 -> MATLAB Function14/3(Mu_current), To Workspace14/1  "Mu_now"
  Add5/1 -> Mu12/1, Radius2/1
  Gain2/1 -> Add5/1
  Mu12/1 -> MATLAB Function14/5(Mu_preview)  "Mu_fut"
  Radius2/1 -> MATLAB Function14/6(Kappa_preview)  "Curv_fut"
  Mu13/1 -> MATLAB Function/9(Mu_in)
  Mu14/1 -> MATLAB Function15/12(Mu_in)
  Gain/1 -> Scope22/1, Gain2/1, Scope21/1, MATLAB Function14/1(Vx_kmh)
  Radius3/1 -> MATLAB Function/10(Curv_in)  "Curv_prev"
  Bus Selector16/1 -> MATLAB Function/11(Delta_f_in)  "<detal_f>"
  Bus Selector26/2 -> MATLAB Function15/11(delta_steering)  "<detal_f>"
  Bus Selector7/2 -> MATLAB Function5/1(Vx)  "<Vx>"
  Bus Selector5/2 -> unitire轮胎力/1(Vx)  "<Vx>"
  Bus Selector8/2 -> MATLAB Function6/1(Vx)  "<Vx>"
  Bus Selector9/2 -> MATLAB Function7/1(Vx)  "<Vx>"
  Bus Selector1/1 -> Bus Creator/1  "<Vx>"
  Bus Selector1/2 -> Bus Creator/2  "<detal_f>"
  Bus Selector26/1 -> MATLAB Function15/2(Vx_act_raw)  "<Vx>"
  [SI] -> MATLAB Function15/15(SI_in)
  Bus Selector26/3 -> MATLAB Function15/14(Beta_in), Radius4/1  "<Beta>"
  Radius4/1 -> MATLAB Function15/13(Curv_in)  "Curv_prev"
  Bus Selector27/2 -> MATLAB Function19/1(Beta)  "<Beta>"
  Radius1/1 -> MATLAB Function14/4(Kappa_current)  "Curv_now"
  Bus Selector15/1 -> Gain/1  "<Vx>"
  Vx2/1 -> MATLAB Function14/2(Vref_kmh)
  Constant63/1 -> Mux10/1
  Constant64/1 -> Mux10/2
  Constant69/1 -> Mux10/3
  Constant71/1 -> Mux10/4
  Constant72/1 -> Mux10/5
  Mux10/1 -> MATLAB Function/6(NN_Weights)
  Vx1/1 -> MATLAB Function18/1(Vx_target_input)
  Bus Selector27/5 -> MATLAB Function19/5(delta_f)  "<detal_f>"

== matlab function siWDqudong_FAN_MPC/Subsystem1/MATLAB Function3 ==
  data: T_total_req input; T_ref_fl output; w_fl input; w_fr input; w_rl input; w_rr input; Fz_fl input; T_ref_fr output; Fz_fr input; Fz_rl input; Fz_rr input; Ay_in input; SI_in input; Mu_in input; Lat_Error_in input; MotorData parameter; T_motor_max input; T_ref_rl output; T_ref_rr output; Mode_Out output; dt input; Debug_Info output
function [T_ref_fl, T_ref_fr, T_ref_rl, T_ref_rr, Mode_Out, Debug_Info] = ...
    Upper_Layer_Optimization_Based(T_total_req, w_fl, w_fr, w_rl, w_rr, ...
    Fz_fl, Fz_fr, Fz_rl, Fz_rr, ...
    Ay_in, SI_in, Mu_in, Lat_Error_in, ...
    MotorData, T_motor_max, dt)
%#codegen
% =========================================================================
% 上层控制器 Anti-Chatter v2
% 物理安全可行域 + 低频能量优化 + 安全域滞回 + lambda速率限制
%
% 直接替换原 Upper_Layer_Optimization_Based。
% 输入/输出接口保持不变。
%
% 主要修正：
% 1) 不再每10 ms用瞬时Ay/Fz直接重算并硬切换lambda；
% 2) Ay、mu、Fz、安全转矩容量全部采用“危险方向快、恢复方向慢”滤波；
% 3) 上层能量优化频率降为20 Hz（50 ms一次），下层MPC仍100 Hz；
% 4) lambda有真正的变化率限制；
% 5) 若当前lambda已经越出物理安全域，则安全投影可以立即覆盖速率限制；
% 6) 新lambda至少带来20 W以上收益才切换，避免追逐效率图微小差异；
% 7) 最终左右轮按平滑Fz比例分配，不再由瞬时Fz造成100 Hz毛刺；
% 8) 若总需求超过当前安全纵向能力，先缩总需求，再做lambda优化；
% 9) 单轮clamp仅保留数值保护，正常情况下不应频繁触发。
% =========================================================================

%% 0. 常数
Re = 0.347;
m  = 1810.0;
lf = 1.152;
lr = 1.528;
L  = lf + lr;

gamma_mu = 0.95;         % 上层安全余量
Ts_upper = 0.05;         % 20 Hz upper optimization
lambda_rate_max = 0.50;  % 1/s
P_improve_min_kW = 0.020;% 至少改善20 W才允许性能型切换
W_lambda_kW = 1.0;       % lambda切换正则，单位kW尺度
num_grid = 31;

%% 1. persistent
persistent last_lambda
persistent T_req_f
persistent upper_timer
persistent Ay_safe_f Mu_safe_f
persistent Fz_alloc_fl Fz_alloc_fr Fz_alloc_rl Fz_alloc_rr
persistent Fz_safe_fl Fz_safe_fr Fz_safe_rl Fz_safe_rr
persistent Tcap_fl_f Tcap_fr_f Tcap_rl_f Tcap_rr_f
persistent map_x_vec map_y_vec map_z_mat
persistent is_initialized

coder.varsize('map_x_vec',[1,5000],[0,1]);
coder.varsize('map_y_vec',[1,5000],[0,1]);
coder.varsize('map_z_mat',[5000,5000],[1,1]);

dt_s = double(dt);
if dt_s <= 0
    dt_s = 0.01;
end

Fz_floor = 100.0;

Fz_fl_raw = max(double(Fz_fl), Fz_floor);
Fz_fr_raw = max(double(Fz_fr), Fz_floor);
Fz_rl_raw = max(double(Fz_rl), Fz_floor);
Fz_rr_raw = max(double(Fz_rr), Fz_floor);

Ay_raw = abs(double(Ay_in(1)));
Mu_raw = min(max(double(Mu_in(1)),0.15),1.20);

if isempty(is_initialized)
    last_lambda = 0.5;
    T_req_f = double(T_total_req(1));
    upper_timer = 0.0;

    Ay_safe_f = Ay_raw;
    Mu_safe_f = Mu_raw;

    Fz_alloc_fl = Fz_fl_raw;
    Fz_alloc_fr = Fz_fr_raw;
    Fz_alloc_rl = Fz_rl_raw;
    Fz_alloc_rr = Fz_rr_raw;

    Fz_safe_fl = Fz_fl_raw;
    Fz_safe_fr = Fz_fr_raw;
    Fz_safe_rl = Fz_rl_raw;
    Fz_safe_rr = Fz_rr_raw;

    Tcap_fl_f = 0.0;
    Tcap_fr_f = 0.0;
    Tcap_rl_f = 0.0;
    Tcap_rr_f = 0.0;

    % 读取效率图
    raw_x = [0,100,200];
    raw_y = [-200,0,200];
    raw_z = 0.90*ones(3,3);

    if ~isempty(MotorData)
        if isfield(MotorData,'Speed_Axis')
            raw_x = double(MotorData.Speed_Axis);
        end
        if isfield(MotorData,'Torque_Axis')
            raw_y = double(MotorData.Torque_Axis);
        end
        if isfield(MotorData,'Eff_Map')
            raw_z = double(MotorData.Eff_Map);
        end
    end

    map_x_vec = reshape(raw_x,1,[]);
    map_y_vec = reshape(raw_y,1,[]);

    [nr,nc] = size(raw_z);
    len_x = length(map_x_vec);
    len_y = length(map_y_vec);

    % 统一内部Z维度为 [Torque x Speed]
    if nr == len_x && nc == len_y
        map_z_mat = raw_z';
    elseif nr == len_y && nc == len_x
        map_z_mat = raw_z;
    else
        map_z_mat = raw_z;
    end

    is_initialized = true;
end

%% 2. 总需求转矩平滑
T_req_raw = double(T_total_req(1));

tau_T = 0.08;
alpha_T = dt_s/(tau_T + dt_s);
T_req_f = T_req_f + alpha_T*(T_req_raw - T_req_f);

%% 3. 平滑用于“名义分配”的Fz
% 这里故意比安全约束慢，避免左右轮名义参考随100 Hz载荷细小波动抖动。
tau_Fz_alloc = 0.12;
alpha_Fz_alloc = dt_s/(tau_Fz_alloc + dt_s);

Fz_alloc_fl = Fz_alloc_fl + alpha_Fz_alloc*(Fz_fl_raw - Fz_alloc_fl);
Fz_alloc_fr = Fz_alloc_fr + alpha_Fz_alloc*(Fz_fr_raw - Fz_alloc_fr);
Fz_alloc_rl = Fz_alloc_rl + alpha_Fz_alloc*(Fz_rl_raw - Fz_alloc_rl);
Fz_alloc_rr = Fz_alloc_rr + alpha_Fz_alloc*(Fz_rr_raw - Fz_alloc_rr);

FzF_alloc = Fz_alloc_fl + Fz_alloc_fr;
FzR_alloc = Fz_alloc_rl + Fz_alloc_rr;

pf_fl = Fz_alloc_fl/max(FzF_alloc,1.0);
pf_fr = Fz_alloc_fr/max(FzF_alloc,1.0);
pr_rl = Fz_alloc_rl/max(FzR_alloc,1.0);
pr_rr = Fz_alloc_rr/max(FzR_alloc,1.0);

%% 4. 危险量采用“危险方向快，恢复方向慢”
% 4.1 Ay：Ay升高=危险，快速；Ay降低=恢复，慢速
Ay_safe_f = asym_filter(Ay_safe_f, Ay_raw, dt_s, 0.035, 0.30, true);

% 4.2 mu：mu降低=危险，快速；mu升高=恢复，慢速
Mu_safe_f = asym_filter(Mu_safe_f, Mu_raw, dt_s, 0.030, 0.40, false);
Mu_safe_f = min(max(Mu_safe_f,0.15),1.20);

% 4.3 Fz：Fz降低=危险，快速；Fz升高=恢复，慢速
Fz_safe_fl = asym_filter(Fz_safe_fl, Fz_fl_raw, dt_s, 0.025, 0.25, false);
Fz_safe_fr = asym_filter(Fz_safe_fr, Fz_fr_raw, dt_s, 0.025, 0.25, false);
Fz_safe_rl = asym_filter(Fz_safe_rl, Fz_rl_raw, dt_s, 0.025, 0.25, false);
Fz_safe_rr = asym_filter(Fz_safe_rr, Fz_rr_raw, dt_s, 0.025, 0.25, false);

%% 5. 估计横向需求
% 仍保持现有接口，不新增四轮Fy端口。
Fy_f_req = m*Ay_safe_f*(lr/L);
Fy_r_req = m*Ay_safe_f*(lf/L);

% 横向力分配采用平滑Fz比例，避免瞬时载荷比例造成左右轮容量跳变
Fy_fl_hat = Fy_f_req*pf_fl;
Fy_fr_hat = Fy_f_req*pf_fr;
Fy_rl_hat = Fy_r_req*pr_rl;
Fy_rr_hat = Fy_r_req*pr_rr;

%% 6. 单轮原始安全纵向能力
T_motor_lim = max(min(abs(double(T_motor_max(1))),350.0),1.0);

Fx_fl_safe = safe_fx_capacity(Mu_safe_f,Fz_safe_fl,Fy_fl_hat,gamma_mu);
Fx_fr_safe = safe_fx_capacity(Mu_safe_f,Fz_safe_fr,Fy_fr_hat,gamma_mu);
Fx_rl_safe = safe_fx_capacity(Mu_safe_f,Fz_safe_rl,Fy_rl_hat,gamma_mu);
Fx_rr_safe = safe_fx_capacity(Mu_safe_f,Fz_safe_rr,Fy_rr_hat,gamma_mu);

Tcap_fl_raw = min(T_motor_lim,Re*Fx_fl_safe);
Tcap_fr_raw = min(T_motor_lim,Re*Fx_fr_safe);
Tcap_rl_raw = min(T_motor_lim,Re*Fx_rl_safe);
Tcap_rr_raw = min(T_motor_lim,Re*Fx_rr_safe);

% 第一次初始化时直接置为真实容量
if Tcap_fl_f <= 0.0 && Tcap_fr_f <= 0.0 && Tcap_rl_f <= 0.0 && Tcap_rr_f <= 0.0
    Tcap_fl_f = Tcap_fl_raw;
    Tcap_fr_f = Tcap_fr_raw;
    Tcap_rl_f = Tcap_rl_raw;
    Tcap_rr_f = Tcap_rr_raw;
else
    % 容量下降=危险，快速；容量恢复=慢速
    Tcap_fl_f = asym_filter(Tcap_fl_f,Tcap_fl_raw,dt_s,0.020,0.25,false);
    Tcap_fr_f = asym_filter(Tcap_fr_f,Tcap_fr_raw,dt_s,0.020,0.25,false);
    Tcap_rl_f = asym_filter(Tcap_rl_f,Tcap_rl_raw,dt_s,0.020,0.25,false);
    Tcap_rr_f = asym_filter(Tcap_rr_f,Tcap_rr_raw,dt_s,0.020,0.25,false);
end

Tcap_fl = max(Tcap_fl_f,0.0);
Tcap_fr = max(Tcap_fr_f,0.0);
Tcap_rl = max(Tcap_rl_f,0.0);
Tcap_rr = max(Tcap_rr_f,0.0);

%% 7. 同轴总能力：必须与最终Fz比例分配一致
Tf_cap = min( ...
    Tcap_fl/max(pf_fl,1e-6), ...
    Tcap_fr/max(pf_fr,1e-6));

Tr_cap = min( ...
    Tcap_rl/max(pr_rl,1e-6), ...
    Tcap_rr/max(pr_rr,1e-6));

Tf_cap = max(Tf_cap,0.0);
Tr_cap = max(Tr_cap,0.0);

%% 8. 先限制“总需求”，再推导lambda安全域
T_total_cap = Tf_cap + Tr_cap;

if abs(T_req_f) <= T_total_cap
    T_req_safe = T_req_f;
else
    T_req_safe = sign_nonzero(T_req_f)*T_total_cap;
end

T_abs = abs(T_req_safe);

if T_abs < 1e-8
    l_min = 0.0;
    l_max = 1.0;
else
    l_min = max(0.0, 1.0 - Tr_cap/(T_abs + 1e-9));
    l_max = min(1.0, Tf_cap/(T_abs + 1e-9));

    if l_min > l_max
        % 数值退化时按能力比例形成唯一点
        cap_sum = Tf_cap + Tr_cap;
        if cap_sum > 1e-9
            l_only = Tf_cap/cap_sum;
        else
            l_only = 0.5;
        end
        l_min = clamp(l_only,0.0,1.0);
        l_max = l_min;
    end
end

%% 9. 安全投影优先
safety_override = 0.0;

if last_lambda < l_min
    last_lambda = l_min;
    safety_override = 1.0;
elseif last_lambda > l_max
    last_lambda = l_max;
    safety_override = 1.0;
end

%% 10. 20 Hz能量优化
upper_timer = upper_timer + dt_s;

if upper_timer >= Ts_upper
    upper_timer = upper_timer - Ts_upper;

    lambda_current = clamp(last_lambda,l_min,l_max);

    J_current = evaluate_lambda_cost( ...
        lambda_current,T_req_safe, ...
        pf_fl,pf_fr,pr_rl,pr_rr, ...
        w_fl,w_fr,w_rl,w_rr, ...
        map_x_vec,map_y_vec,map_z_mat, ...
        last_lambda,W_lambda_kW);

    best_lambda = lambda_current;
    best_cost = J_current;

    if l_max > l_min
        step_lambda = (l_max-l_min)/(num_grid-1);
    else
        step_lambda = 0.0;
    end

    for kk = 0:num_grid-1
        lambda_c = l_min + kk*step_lambda;

        J_c = evaluate_lambda_cost( ...
            lambda_c,T_req_safe, ...
            pf_fl,pf_fr,pr_rl,pr_rr, ...
            w_fl,w_fr,w_rl,w_rr, ...
            map_x_vec,map_y_vec,map_z_mat, ...
            last_lambda,W_lambda_kW);

        if J_c < best_cost
            best_cost = J_c;
            best_lambda = lambda_c;
        end
    end

    % 只有收益达到最小阈值才执行“性能型切换”
    improvement_kW = J_current - best_cost;

    if improvement_kW >= P_improve_min_kW
        lambda_target = best_lambda;
    else
        lambda_target = lambda_current;
    end

    % 性能调节受lambda速率限制
    d_lambda_max = lambda_rate_max*Ts_upper;
    d_lambda = lambda_target - last_lambda;
    d_lambda = clamp(d_lambda,-d_lambda_max,d_lambda_max);

    lambda_new = last_lambda + d_lambda;

    % 再投影回安全域
    lambda_new = clamp(lambda_new,l_min,l_max);

    last_lambda = lambda_new;
end

%% 11. 最终四轮名义参考
lambda_cmd = clamp(last_lambda,l_min,l_max);

Front_Tot = T_req_safe*lambda_cmd;
Rear_Tot  = T_req_safe*(1.0-lambda_cmd);

T_ref_fl = Front_Tot*pf_fl;
T_ref_fr = Front_Tot*pf_fr;
T_ref_rl = Rear_Tot*pr_rl;
T_ref_rr = Rear_Tot*pr_rr;

% 仅做数值保护；按上面的轴能力推导，正常情况下不会频繁触发
T_ref_fl = clamp(T_ref_fl,-Tcap_fl,Tcap_fl);
T_ref_fr = clamp(T_ref_fr,-Tcap_fr,Tcap_fr);
T_ref_rl = clamp(T_ref_rl,-Tcap_rl,Tcap_rl);
T_ref_rr = clamp(T_ref_rr,-Tcap_rr,Tcap_rr);

%% 12. Debug
SI_val = double(SI_in(1));
Lat_val = abs(double(Lat_Error_in(1)));

R_Ay = max(0.0,(Ay_safe_f/(Mu_safe_f*9.81+0.1))-0.7)/0.3;
R_SI = clamp((SI_val-0.5)/0.4,0.0,1.0);
R_Lat = clamp((Lat_val-0.5)/0.5,0.0,1.0);
Risk_Factor = max([R_Ay,R_SI,R_Lat]);

Mode_Out = 1.0-lambda_cmd;

% Debug:
% 1 lambda_cmd
% 2 lambda_min
% 3 lambda_max
% 4 T_req_safe
% 5 Risk_Factor
Debug_Info = [lambda_cmd;l_min;l_max;T_req_safe;Risk_Factor];

end

%% ================= local functions =================

function y = asym_filter(y_prev, x_now, dt, tau_danger, tau_recover, danger_is_increase)
% 危险方向快，恢复方向慢
    if danger_is_increase
        is_danger = x_now > y_prev;
    else
        is_danger = x_now < y_prev;
    end

    if is_danger
        tau = tau_danger;
    else
        tau = tau_recover;
    end

    alpha = dt/(tau + dt);
    alpha = min(max(alpha,0.0),1.0);

    y = y_prev + alpha*(x_now-y_prev);
end

function Fx_safe = safe_fx_capacity(mu,Fz,Fy_hat,gamma_mu)
    Ftot = gamma_mu*mu*Fz;
    Fx_safe = sqrt(max(Ftot*Ftot - Fy_hat*Fy_hat,0.0));
end

function JkW = evaluate_lambda_cost(lambda,Treq, ...
    pf_fl,pf_fr,pr_rl,pr_rr, ...
    w_fl,w_fr,w_rl,w_rr, ...
    x_axis,y_axis,z_map,lambda_prev,W_lambda_kW)

    Tf = lambda*Treq;
    Tr = (1.0-lambda)*Treq;

    Tfl = Tf*pf_fl;
    Tfr = Tf*pf_fr;
    Trl = Tr*pr_rl;
    Trr = Tr*pr_rr;

    P_batt = ...
        calc_battery_power(Tfl,abs(double(w_fl)),x_axis,y_axis,z_map) + ...
        calc_battery_power(Tfr,abs(double(w_fr)),x_axis,y_axis,z_map) + ...
        calc_battery_power(Trl,abs(double(w_rl)),x_axis,y_axis,z_map) + ...
        calc_battery_power(Trr,abs(double(w_rr)),x_axis,y_axis,z_map);

    J_switch = W_lambda_kW*(lambda-lambda_prev)^2;

    JkW = P_batt/1000.0 + J_switch;
end

function P_batt = calc_battery_power(T_val,w_val,x_axis,y_axis,z_map)
    if abs(T_val) < 0.05 || abs(w_val) < 1e-6
        P_batt = 0.0;
        return;
    end

    if y_axis(1) < -1e-6
        tq_query = T_val;
    else
        tq_query = abs(T_val);
    end

    eff = manual_bilinear_interp(x_axis,y_axis,z_map,abs(w_val),tq_query);
    eff = max(min(eff,0.98),0.05);

    P_mech = T_val*abs(w_val);

    if P_mech >= 0.0
        P_batt = P_mech/eff;
    else
        P_batt = P_mech*eff;
    end
end

function val = manual_bilinear_interp(X,Y,Z,xq,yq)
    xq = max(min(xq,X(end)),X(1));
    yq = max(min(yq,Y(end)),Y(1));

    idx_x = 1;
    for k = 1:length(X)-1
        if xq >= X(k) && xq <= X(k+1)
            idx_x = k;
            break;
        end
    end
    if idx_x >= length(X)
        idx_x = length(X)-1;
    end

    idx_y = 1;
    for k = 1:length(Y)-1
        if yq >= Y(k) && yq <= Y(k+1)
            idx_y = k;
            break;
        end
    end
    if idx_y >= length(Y)
        idx_y = length(Y)-1;
    end

    dx = X(idx_x+1)-X(idx_x);
    dy = Y(idx_y+1)-Y(idx_y);

    u = (xq-X(idx_x))/(dx+1e-9);
    v = (yq-Y(idx_y))/(dy+1e-9);

    z11 = Z(idx_y,idx_x);
    z12 = Z(idx_y,idx_x+1);
    z21 = Z(idx_y+1,idx_x);
    z22 = Z(idx_y+1,idx_x+1);

    val = (1-v)*((1-u)*z11 + u*z12) + ...
           v*((1-u)*z21 + u*z22);
end

function y = clamp(x,lo,hi)
    y = max(min(x,hi),lo);
end

function s = sign_nonzero(x)
    if x >= 0
        s = 1.0;
    else
        s = -1.0;
    end
end

== matlab function siWDqudong_FAN_MPC/Subsystem1/MATLAB Function4 ==
  data: Vx input; beta_ref output; delta_f input; lf input; lr input; Kyf input; Kyr input; m input; dt input
function beta_ref = Beta_Ref_Generation_Constant(Vx, delta_f, lf, lr, Kyf, Kyr, m, dt)
% =========================================================================
% 质心侧偏角参考值生成 (终极数学修正版)
% 修复：原公式量纲错误，现替换为严谨的 2DOF 稳态响应物理公式
% =========================================================================
    % 1. 输入预处理
    Vx_safe = max(abs(Vx), 1.0) * sign(Vx); % 避免低速奇异
    L = lf + lr;

    % 2. 转换为整轴侧偏刚度 (极度重要)
    Kyf_axle = Kyf * 2; 
    Kyr_axle = Kyr * 2;

    % 3. 计算稳态横摆增益 Ks 
    % 注意：因为已经用了整轴刚度，公式分母是 L^2 而不是 2L^2
    K_s = (m / L^2) * (lr / Kyf_axle - lf / Kyr_axle);

    % 4. 使用正确的稳态质心侧偏角公式
    % 公式: beta = delta * (lr - lf*m*Vx^2 / (Kyr_axle*L)) / (L * (1 + Ks*Vx^2))
    term_num = lr - (lf * m * Vx_safe^2) / (Kyr_axle * L);
    term_den = L * (1 + K_s * Vx_safe^2);
    
    beta_ref_raw = (term_num / term_den) * delta_f;

    % 5. 低通滤波 (模拟真实车辆惯性延迟，必须保留！)
    persistent beta_prev;
    if isempty(beta_prev)
        beta_prev = 0;
    end
    tau = 0.05;
    beta_smoothed = (dt * beta_ref_raw + tau * beta_prev) / (tau + dt);

    % 6. 幅值限制
    beta_max = 8 * pi / 180;
    beta_ref = max(min(beta_smoothed, beta_max), -beta_max);

    % 更新历史值
    beta_prev = beta_ref;
    beta_ref = real(beta_ref);
end
